simulink model "SRI_Flu_Epidemic_Model"  (R2025a)
settings: Solver=VariableStepAuto  StartTime=0.0  StopTime=1209600  RelTol=1e-3
undefined symbols (not defined in the file): a, r
settings Model: Creator=demarcewilliams  LastModifiedBy=demarcewilliams

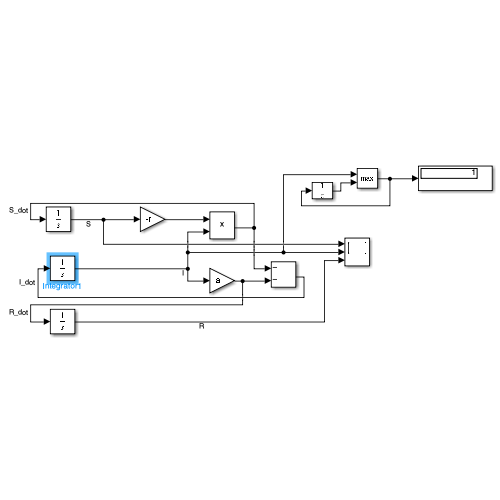
[thumbnail: Simulink's stored preview of the top-level diagram]
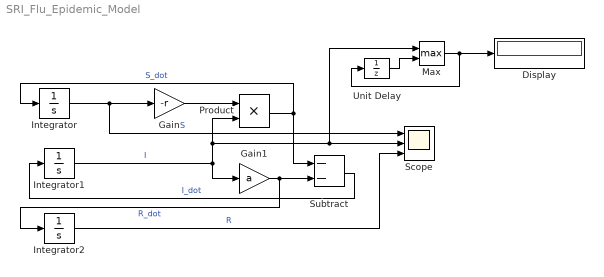
== system SRI_Flu_Epidemic_Model ==
  Display : Display
  Gain : Gain  Gain=-r
  Gain1 : Gain  Gain=a
  Integrator : Integrator  InitialCondition=999
  Integrator1 : Integrator  InitialCondition=1
  Integrator2 : Integrator
  Max : MinMax  Function=max  Inputs=2
  Product : Product
  Scope : Scope  NumInputPorts=3
      settings: ActiveDisplayYMinimum=-0.044551807281332456  ActiveDisplayYMaximum=0.27892480774192452
  Subtract : Sum  Inputs=--
  Unit Delay : UnitDelay  SampleTime=-1  HasFrameUpgradeWarning=on
  wires:
  Product/1 -> Subtract/1, Integrator/1  "S_dot"
  Subtract/1 -> Integrator1/1  "I_dot"
  Gain1/1 -> Integrator2/1, Subtract/2  "R_dot"
  Integrator/1 -> Scope/1, Gain/1  "S"
  Integrator1/1 -> Gain1/1, Product/2, Max/1, Scope/2  "I"
  Integrator2/1 -> Scope/3  "R"
  Gain/1 -> Product/1
  Max/1 -> Display/1, Unit Delay/1
  Unit Delay/1 -> Max/2
